simulink model "Delt_Effivtive"  (R2018b)
settings: Solver=VariableStepAuto  StartTime=0.0  StopTime=10.0  RelTol=1e-3
settings Model: Creator=auten  LastModifiedBy=auten

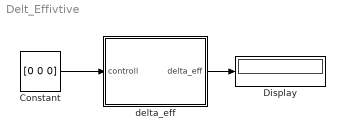
== system Delt_Effivtive ==
  Constant : Constant  Value=[0 0 0]  VectorParams1D=off  SampleTime=-1
  Display : Display
  delta_eff : Subsystem
  wires:
  Constant/1 -> delta_eff/1(controll)
  delta_eff/1(delta_eff) -> Display/1

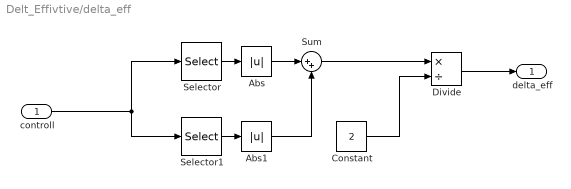
== system Delt_Effivtive/delta_eff ==
  controll : Inport
  Abs : Abs
  Abs1 : Abs
  Constant : Constant  Value=2
  Divide : Product  Inputs=*/  SaturateOnIntegerOverflow=on  RndMeth=Zero
  Selector : Selector  InputPortWidth=3  IndexOptions=Index vector (dialog)  Indices=[3]  OutputSizes=1
  Selector1 : Selector  InputPortWidth=3  IndexOptions=Index vector (dialog)  Indices=[2]  OutputSizes=1
  Sum : Sum  Inputs=|++
  delta_eff : Outport
  wires:
  Selector1/1 -> Abs1/1
  Sum/1 -> Divide/1
  Constant/1 -> Divide/2
  Divide/1 -> delta_eff/1
  controll/1 -> Selector/1, Selector1/1
  Selector/1 -> Abs/1
  Abs/1 -> Sum/1
  Abs1/1 -> Sum/2
